simulink model "Task_Space_Centralized_Control_Feedback_Linearization"  (R2024a)
settings: Solver=VariableStepAuto  StartTime=0.0  StopTime=10  RelTol=1e-3
settings Model: Creator=ANDALIBM  LastModifiedBy=kaviarasu
settings DataIOCC: ReturnWorkspaceOutputs=off
settings DebuggingCC: UnconnectedInputMsg=warning  UnconnectedOutputMsg=warning  UnconnectedLineMsg=warning
settings ModelReferenceCC: EnableRefExpFcnMdlSchedulingChecks=on
settings RTWCC: GPUComputeCapability=3.5  DLArmComputeVersion=19.05

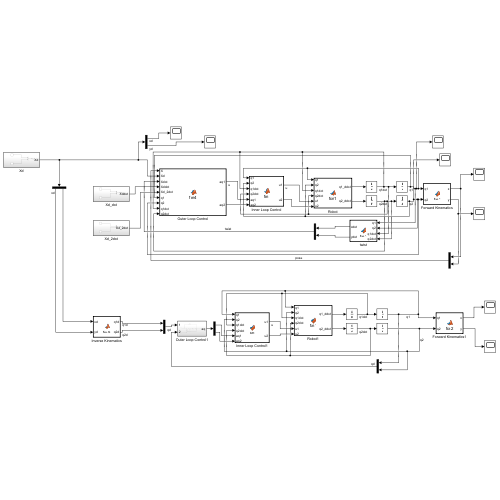
[thumbnail: Simulink's stored preview of the top-level diagram]
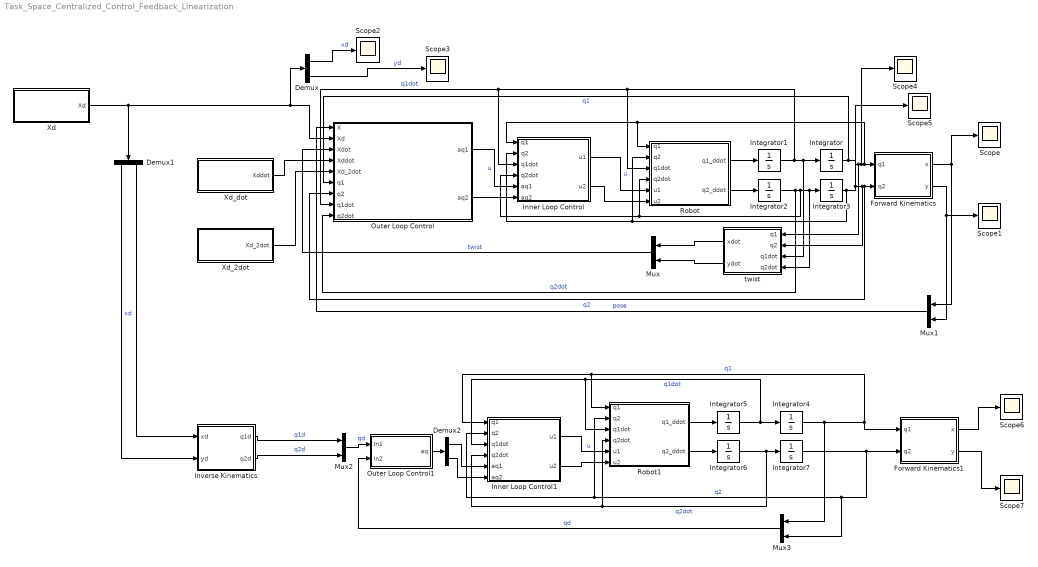
== system Task_Space_Centralized_Control_Feedback_Linearization ==
  Demux : Demux  Outputs=2
  Demux1 : Demux  Outputs=2
  Demux2 : Demux  Outputs=2
  Forward Kinematics : MATLAB Function  TreatAsAtomicUnit=on
  Forward Kinematics1 : MATLAB Function  TreatAsAtomicUnit=on
  Inner Loop Control : MATLAB Function  TreatAsAtomicUnit=on
  Inner Loop Control1 : MATLAB Function  TreatAsAtomicUnit=on
  Integrator : Integrator  InitialCondition=pi/30
  Integrator{1..2,5..6} (4 alike) : Integrator
  Integrator3 : Integrator  InitialCondition=pi/18
  Integrator4 : Integrator  InitialCondition=pi/30
  Integrator7 : Integrator  InitialCondition=pi/18
  Inverse Kinematics : MATLAB Function  TreatAsAtomicUnit=on
  Mux{,1..3} (4 alike) : Mux  Inputs=2
  Outer Loop Control : MATLAB Function  TreatAsAtomicUnit=on
  Outer Loop Control1 : Subsystem
  Robot : MATLAB Function  TreatAsAtomicUnit=on
  Robot1 : MATLAB Function  TreatAsAtomicUnit=on
  Scope{,1..7} (8 alike) : Scope
  Xd : Subsystem
  Xd_2dot : Subsystem
  Xd_dot : Subsystem
  twist : MATLAB Function  TreatAsAtomicUnit=on
  wires:
  Robot/1(q1_ddot) -> Integrator1/1
  Integrator1/1 -> Robot/3(q1dot), Inner Loop Control/3(q1dot), Outer Loop Control/8(q1dot), twist/3(q1dot), Integrator/1  "q1dot"
  Integrator2/1 -> Outer Loop Control/9(q2dot), Robot/4(q2dot), Inner Loop Control/4(q2dot), twist/4(q2dot), Integrator3/1  "q2dot"
  Robot/2(q2_ddot) -> Integrator2/1
  Integrator/1 -> Outer Loop Control/6(q1), twist/1(q1), Scope4/1, Robot/1(q1), Inner Loop Control/1(q1), Forward Kinematics/1(q1)  "q1"
  Integrator3/1 -> Robot/2(q2), Inner Loop Control/2(q2), Scope5/1, twist/2(q2), Outer Loop Control/7(q2), Forward Kinematics/2(q2)  "q2"
  Forward Kinematics/1(x) -> Scope/1, Mux1/1
  Forward Kinematics/2(y) -> Mux1/2, Scope1/1
  twist/1(xdot) -> Mux/1
  twist/2(ydot) -> Mux/2
  Xd/1(Xd) -> Demux1/1, Demux/1, Outer Loop Control/2(Xd)
  Xd_dot/1(Xddot) -> Outer Loop Control/4(Xddot)
  Xd_2dot/1(Xd_2dot) -> Outer Loop Control/5(Xd_2dot)
  Mux1/1 -> Outer Loop Control/1(X)  "pose"
  Mux/1 -> Outer Loop Control/3(Xdot)  "twist"
  Outer Loop Control/1(aq1) -> Inner Loop Control/5(aq1)  "u"
  Outer Loop Control/2(aq2) -> Inner Loop Control/6(aq2)
  Inner Loop Control/1(u1) -> Robot/5(u1)  "u"
  Inner Loop Control/2(u2) -> Robot/6(u2)
  Demux/1 -> Scope2/1  "xd"
  Demux/2 -> Scope3/1  "yd"
  Inverse Kinematics/2(q2d) -> Mux2/2  "q2d"
  Robot1/2(q2_ddot) -> Integrator6/1
  Inverse Kinematics/1(q1d) -> Mux2/1  "q1d"
  Integrator5/1 -> Robot1/3(q1dot), Inner Loop Control1/3(q1dot), Integrator4/1  "q1dot"
  Robot1/1(q1_ddot) -> Integrator5/1
  Integrator7/1 -> Mux3/2, Robot1/2(q2), Inner Loop Control1/2(q2), Forward Kinematics1/2(q2)  "q2"
  Mux3/1 -> Outer Loop Control1/2(In2)  "qd"
  Integrator6/1 -> Robot1/4(q2dot), Inner Loop Control1/4(q2dot), Integrator7/1  "q2dot"
  Inner Loop Control1/2(u2) -> Robot1/6(u2)
  Mux2/1 -> Outer Loop Control1/1(In1)  "qd"
  Demux2/2 -> Inner Loop Control1/6(aq2)
  Outer Loop Control1/1(aq) -> Demux2/1
  Demux2/1 -> Inner Loop Control1/5(aq1)
  Inner Loop Control1/1(u1) -> Robot1/5(u1)  "u"
  Integrator4/1 -> Mux3/1, Robot1/1(q1), Inner Loop Control1/1(q1), Forward Kinematics1/1(q1)  "q1"
  Demux1/2 -> Inverse Kinematics/1(xd)
  Forward Kinematics1/1(x) -> Scope6/1
  Forward Kinematics1/2(y) -> Scope7/1
  Demux1/1 -> Inverse Kinematics/2(yd)  "xd"

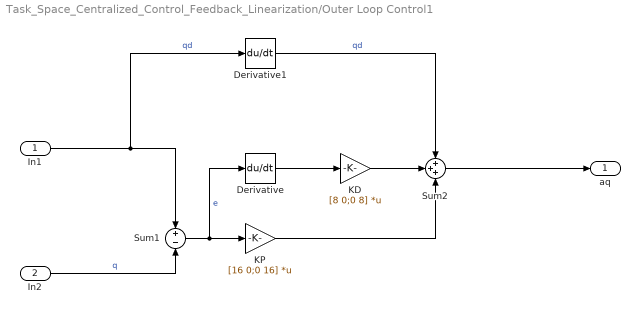
== system Task_Space_Centralized_Control_Feedback_Linearization/Outer Loop Control1 ==
  In1 : Inport
  In2 : Inport  Port=2
  Derivative : Derivative
  Derivative1 : Derivative
  KD : Gain  Gain=[8 0;0 8]  Multiplication=Matrix(K*u)
  KP : Gain  Gain=[16 0;0 16]  Multiplication=Matrix(K*u)
  Sum1 : Sum  Inputs=+-
  Sum2 : Sum  Inputs=+++
  aq : Outport
  wires:
  KD/1 -> Sum2/2
  KP/1 -> Sum2/3
  Sum1/1 -> Derivative/1, KP/1  "e"
  Derivative/1 -> KD/1
  In1/1 -> Derivative1/1, Sum1/1  "qd"
  In2/1 -> Sum1/2  "q"
  Sum2/1 -> aq/1
  Derivative1/1 -> Sum2/1  "qd"

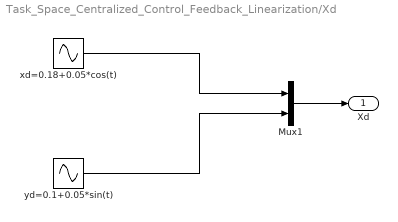
== system Task_Space_Centralized_Control_Feedback_Linearization/Xd ==
  Mux1 : Mux  Inputs=2
  xd=0.18+0.05*cos(t) : Sin  Amplitude=0.05  Bias=0.18  Phase=pi/2  SampleTime=0
  yd=0.1+0.05*sin(t) : Sin  Amplitude=0.05  Bias=0.1  SampleTime=0
  Xd : Outport
  wires:
  Mux1/1 -> Xd/1
  xd=0.18+0.05*cos(t)/1 -> Mux1/1
  yd=0.1+0.05*sin(t)/1 -> Mux1/2

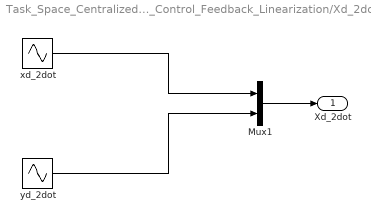
== system Task_Space_Centralized_Control_Feedback_Linearization/Xd_2dot ==
  Mux1 : Mux  Inputs=2
  xd_2dot : Sin  Amplitude=0.05  Phase=3*pi/2  SampleTime=0
  yd_2dot : Sin  Amplitude=0.05  Phase=pi  SampleTime=0
  Xd_2dot : Outport
  wires:
  yd_2dot/1 -> Mux1/2
  xd_2dot/1 -> Mux1/1
  Mux1/1 -> Xd_2dot/1

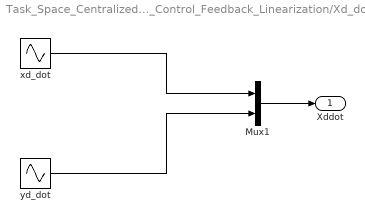
== system Task_Space_Centralized_Control_Feedback_Linearization/Xd_dot ==
  Mux1 : Mux  Inputs=2
  xd_dot : Sin  Amplitude=0.05  Phase=pi  SampleTime=0
  yd_dot : Sin  Amplitude=0.05  Phase=pi/2  SampleTime=0
  Xddot : Outport
  wires:
  Mux1/1 -> Xddot/1
  xd_dot/1 -> Mux1/1
  yd_dot/1 -> Mux1/2

== matlab function Task_Space_Centralized_Control_Feedback_Linearization/Inverse Kinematics ==
  data: xd input; q1d output; yd input; q2d output
function [q1d,q2d] = fcn5(xd,yd)

a1=0.2;  
a2=0.12; 

D=(a1^2+a2^2-xd^2-yd^2)/(2*a1*a2);
q2d=atan2(sqrt(1-D^2),D);
q1d=atan2(yd,xd)-atan2(a2*sin(q2d),a1+a2*cos(q2d));

== matlab function Task_Space_Centralized_Control_Feedback_Linearization/Forward Kinematics1 ==
  data: q1 input; x output; q2 input; y output
function [x,y] = fcn2(q1,q2)

a1=0.2;  
a2=0.12; 

x=a1*cos(q1)+a2*cos(q1+q2);
y=a1*sin(q1)+a2*sin(q1+q2);

== matlab function Task_Space_Centralized_Control_Feedback_Linearization/Robot ==
  data: q1 input; q1_ddot output; q2 input; q1dot input; q2dot input; u1 input; u2 input; q2_ddot output
function [q1_ddot,q2_ddot] = fcn1(q1,q2,q1dot,q2dot,u1,u2)

g=9.81;
a1=0.2;  
a2=0.12; 
m1=0.4;
m2=0.3;
Im=[0.0016 0.0016];
r1=19.7;
r2=19.7; 
I1=[0 0 0;0 m1*a1^2/12 0;0 0 m1*a1^2/12];
I2=[0 0 0;0 m2*a2^2/12 0;0 0 m2*a2^2/12];
Itot1=I1+r1^2*Im(1); 
Itot2=I2+r2^2*Im(2); 

R1=[cos(q1) -sin(q1) 0;sin(q1) cos(q1) 0;0 0 1];
R2=[cos(q1+q2) -sin(q1+q2) 0;sin(q1+q2) cos(q1+q2) 0;0 0 1];

Jw1=[0 0;0 0;1 0];
Jw2=[0 0;0 0;1 1];
Jv1=[-a1*sin(q1)/2 0;a1*cos(q1)/2 0;0 0];
Jv2=[-a1*sin(q1)-a2*sin(q1+q2)/2 -a2*sin(q1+q2)/2;...
     a1*cos(q1)+a2*cos(q1+q2)/2 a2*cos(q1+q2)/2;...
     0 0];
 
M=(m1*transpose(Jv1)*Jv1+Jw1'*R1*Itot1*R1'*Jw1)+(m2*transpose(Jv2)*Jv2+Jw2'*R2*Itot2*R2'*Jw2);

g1=m1*a1*g*cos(q1)/2+m2*a1*g*cos(q1)+m2*a2*g*cos(q1+q2)/2;
g2=m2*a2*g*cos(q1+q2)/2;
gvec=[g1;g2];

c111=0;
c121=-m2*a1*a2*sin(q2)/2;
c211=c121;
c221=-m2*a1*a2*sin(q2)/2;
c112=m2*a1*a2*sin(q2)/2;
c122=0;
c212=0;
c222=0;

c_qdot=[(c121+c221)*q1dot*q2dot+(c111+c211)*q1dot^2;...
        c112*q1dot^2+(c122+c212)*q1dot*q2dot+c222*q2dot^2];

q2dot = inv(M)*([u1;u2]-c_qdot-gvec);

q1_ddot=q2dot(1);
q2_ddot=q2dot(2);

== matlab function Task_Space_Centralized_Control_Feedback_Linearization/Inner Loop Control ==
  data: q1 input; u1 output; q2 input; q1dot input; q2dot input; aq1 input; aq2 input; u2 output
function [u1,u2] = fcn(q1,q2,q1dot,q2dot,aq1,aq2)

g=9.81;
a1=0.2;  
a2=0.12; 
m1=0.4;
m2=0.3;
Im=[0.0016 0.0016];
r1=19.7;
r2=19.7; 
I1=[0 0 0;0 m1*a1^2/12 0;0 0 m1*a1^2/12];
I2=[0 0 0;0 m2*a2^2/12 0;0 0 m2*a2^2/12];
Itot1=I1+r1^2*Im(1); 
Itot2=I2+r2^2*Im(2); 

R1=[cos(q1) -sin(q1) 0;sin(q1) cos(q1) 0;0 0 1];
R2=[cos(q1+q2) -sin(q1+q2) 0;sin(q1+q2) cos(q1+q2) 0;0 0 1];

Jw1=[0 0;0 0;1 0];
Jw2=[0 0;0 0;1 1];
Jv1=[-a1*sin(q1)/2 0;a1*cos(q1)/2 0;0 0];
Jv2=[-a1*sin(q1)-a2*sin(q1+q2)/2 -a2*sin(q1+q2)/2;...
     a1*cos(q1)+a2*cos(q1+q2)/2 a2*cos(q1+q2)/2;...
     0 0];
 
M=(m1*transpose(Jv1)*Jv1+Jw1'*R1*Itot1*R1'*Jw1)+(m2*transpose(Jv2)*Jv2+Jw2'*R2*Itot2*R2'*Jw2);

g1=m1*a1*g*cos(q1)/2+m2*a1*g*cos(q1)+m2*a2*g*cos(q1+q2)/2;
g2=m2*a2*g*cos(q1+q2)/2;
gvec=[g1;g2];

c111=0;
c121=-m2*a1*a2*sin(q2)/2;
c211=c121;
c221=-m2*a1*a2*sin(q2)/2;
c112=m2*a1*a2*sin(q2)/2;
c122=0;
c212=0;
c222=0;

c_qdot=[(c121+c221)*q1dot*q2dot+(c111+c211)*q1dot^2;...
        c112*q1dot^2+(c122+c212)*q1dot*q2dot+c222*q2dot^2];

u = M*[aq1;aq2]+c_qdot+gvec;

u1=u(1);
u2=u(2);

== matlab function Task_Space_Centralized_Control_Feedback_Linearization/Forward Kinematics ==
  data: q1 input; x output; q2 input; y output
function [x,y] = fcn2(q1,q2)

a1=0.2;  
a2=0.12; 

x=a1*cos(q1)+a2*cos(q1+q2);
y=a1*sin(q1)+a2*sin(q1+q2);

== matlab function Task_Space_Centralized_Control_Feedback_Linearization/twist ==
  data: q1 input; xdot output; q2 input; q1dot input; q2dot input; ydot output
function [xdot,ydot] = fcn3(q1,q2,q1dot,q2dot)

a1=0.2;  
a2=0.12; 

xdot= -a1*sin(q1)*q1dot-a2*sin(q1+q2)*(q1dot+q2dot);
ydot= a1*cos(q1)*q1dot+a2*cos(q1+q2)*(q1dot+q2dot);

== matlab function Task_Space_Centralized_Control_Feedback_Linearization/Outer Loop Control ==
  data: X input; Xd input; Xdot input; Xddot input; Xd_2dot input; q1 input; aq1 output; q2 input; q1dot input; q2dot input; aq2 output
function [aq1,aq2] = fcn4(X,Xd,Xdot,Xddot,Xd_2dot,q1,q2,q1dot,q2dot)

a1=0.2;  
a2=0.12;

Kp=[16 0;0 16];

Kd=[8 0;0 8];

J=[-a1*sin(q1)-a2*sin(q1+q2) -a2*sin(q1+q2);...
    a1*cos(q1)+a2*cos(q1+q2) a2*cos(q1+q2)];

Jdot=[-a1*cos(q1)*q1dot-a2*cos(q1+q2)*(q1dot+q2dot) -a2*cos(q1+q2)*(q1dot+q2dot);...
      -a1*sin(q1)*q1dot-a2*sin(q1+q2)*(q1dot+q2dot) -a2*sin(q1+q2)*(q1dot+q2dot)];

aq=inv(J)*(Xd_2dot+Kp*(Xd-X)+Kd*(Xddot-Xdot)-Jdot*[q1dot;q2dot]);

aq1=aq(1);
aq2=aq(2);

== matlab function Task_Space_Centralized_Control_Feedback_Linearization/Inner Loop Control1 ==
  data: q1 input; u1 output; q2 input; q1dot input; q2dot input; aq1 input; aq2 input; u2 output
function [u1,u2] = fcn(q1,q2,q1dot,q2dot,aq1,aq2)

g=9.81;
a1=0.2;  
a2=0.12; 
m1=0.4;
m2=0.3;
Im=[0.0016 0.0016];
r1=19.7;
r2=19.7; 
I1=[0 0 0;0 m1*a1^2/12 0;0 0 m1*a1^2/12];
I2=[0 0 0;0 m2*a2^2/12 0;0 0 m2*a2^2/12];
Itot1=I1+r1^2*Im(1); 
Itot2=I2+r2^2*Im(2); 

R1=[cos(q1) -sin(q1) 0;sin(q1) cos(q1) 0;0 0 1];
R2=[cos(q1+q2) -sin(q1+q2) 0;sin(q1+q2) cos(q1+q2) 0;0 0 1];

Jw1=[0 0;0 0;1 0];
Jw2=[0 0;0 0;1 1];
Jv1=[-a1*sin(q1)/2 0;a1*cos(q1)/2 0;0 0];
Jv2=[-a1*sin(q1)-a2*sin(q1+q2)/2 -a2*sin(q1+q2)/2;...
     a1*cos(q1)+a2*cos(q1+q2)/2 a2*cos(q1+q2)/2;...
     0 0];
 
M=(m1*transpose(Jv1)*Jv1+Jw1'*R1*Itot1*R1'*Jw1)+(m2*transpose(Jv2)*Jv2+Jw2'*R2*Itot2*R2'*Jw2);

g1=m1*a1*g*cos(q1)/2+m2*a1*g*cos(q1)+m2*a2*g*cos(q1+q2)/2;
g2=m2*a2*g*cos(q1+q2)/2;
gvec=[g1;g2];

c111=0;
c121=-m2*a1*a2*sin(q2)/2;
c211=c121;
c221=-m2*a1*a2*sin(q2)/2;
c112=m2*a1*a2*sin(q2)/2;
c122=0;
c212=0;
c222=0;

c_qdot=[(c121+c221)*q1dot*q2dot+(c111+c211)*q1dot^2;...
        c112*q1dot^2+(c122+c212)*q1dot*q2dot+c222*q2dot^2];

u = M*[aq1;aq2]+c_qdot+gvec;

u1=u(1);
u2=u(2);

== matlab function Task_Space_Centralized_Control_Feedback_Linearization/Robot1 ==
  data: q1 input; q1_ddot output; q2 input; q1dot input; q2dot input; u1 input; u2 input; q2_ddot output
function [q1_ddot,q2_ddot] = fcn1(q1,q2,q1dot,q2dot,u1,u2)

g=9.81;
a1=0.2;  
a2=0.12; 
m1=0.4;
m2=0.3;
Im=[0.0016 0.0016];
r1=19.7;
r2=19.7; 
I1=[0 0 0;0 m1*a1^2/12 0;0 0 m1*a1^2/12];
I2=[0 0 0;0 m2*a2^2/12 0;0 0 m2*a2^2/12];
Itot1=I1+r1^2*Im(1); 
Itot2=I2+r2^2*Im(2); 

R1=[cos(q1) -sin(q1) 0;sin(q1) cos(q1) 0;0 0 1];
R2=[cos(q1+q2) -sin(q1+q2) 0;sin(q1+q2) cos(q1+q2) 0;0 0 1];

Jw1=[0 0;0 0;1 0];
Jw2=[0 0;0 0;1 1];
Jv1=[-a1*sin(q1)/2 0;a1*cos(q1)/2 0;0 0];
Jv2=[-a1*sin(q1)-a2*sin(q1+q2)/2 -a2*sin(q1+q2)/2;...
     a1*cos(q1)+a2*cos(q1+q2)/2 a2*cos(q1+q2)/2;...
     0 0];
 
M=(m1*transpose(Jv1)*Jv1+Jw1'*R1*Itot1*R1'*Jw1)+(m2*transpose(Jv2)*Jv2+Jw2'*R2*Itot2*R2'*Jw2);

g1=m1*a1*g*cos(q1)/2+m2*a1*g*cos(q1)+m2*a2*g*cos(q1+q2)/2;
g2=m2*a2*g*cos(q1+q2)/2;
gvec=[g1;g2];

c111=0;
c121=-m2*a1*a2*sin(q2)/2;
c211=c121;
c221=-m2*a1*a2*sin(q2)/2;
c112=m2*a1*a2*sin(q2)/2;
c122=0;
c212=0;
c222=0;

c_qdot=[(c121+c221)*q1dot*q2dot+(c111+c211)*q1dot^2;...
        c112*q1dot^2+(c122+c212)*q1dot*q2dot+c222*q2dot^2];

q2dot = inv(M)*([u1;u2]-c_qdot-gvec);

q1_ddot=q2dot(1);
q2_ddot=q2dot(2);
